simulink model "Polynomial_model_for_locked_state_1"  (R2025a)
settings: Solver=VariableStepAuto  StartTime=0.0  StopTime=10.0  RelTol=1e-3
values from neighbouring files (symbols this model uses):
  Divider_Controller = 0    [Close_Loop_ENOP_stable.m]
  IC1 = [0 0 0 0]    [Close_Loop_ENOP_stable.m]
  icp_offset = 0    [Close_Loop_ENOP_stable.m]
  inp = 1023    [Close_Loop_ENOP_stable.m]
  LSB_Dither = 1    [Close_Loop_ENOP_stable.m]
  M = 1024^2    (= 1048576)    [Close_Loop_ENOP_stable.m]
  Nint = 45    [Close_Loop_ENOP_stable.m]
libraries: dspobslib x5
settings Model: Creator=haoyang  LastModifiedBy=HaoyangShen

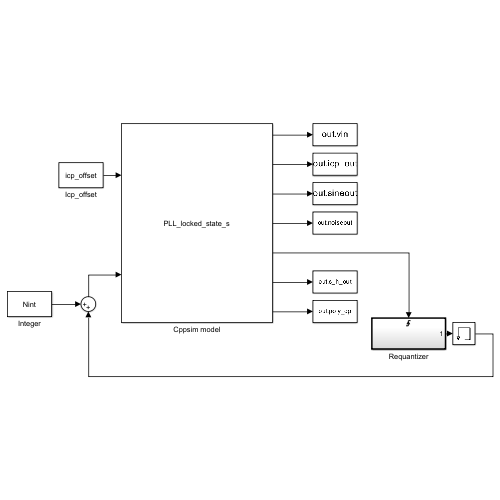
[thumbnail: Simulink's stored preview of the top-level diagram]
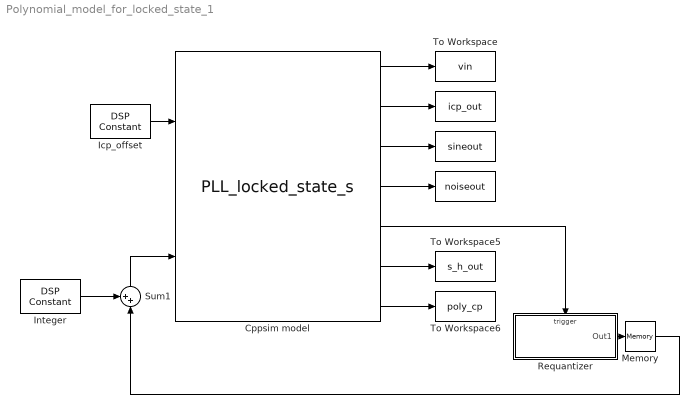
== system Polynomial_model_for_locked_state_1 ==
  " " : ToWorkspace  VariableName=icp_out  SampleTime=-1
  "  " : ToWorkspace  VariableName=sineout  SampleTime=-1
  "   " : ToWorkspace  VariableName=noiseout  SampleTime=-1
  Cppsim model : S-Function  FunctionName=PLL_locked_state_s  Parameters=Ts, pfd_freq, pfd_reset_delay, pfd_down_xdelay, icp, icp_error, icp_thermal_noise_up, icp_thermal_noise_down, icp_flicker_corner_freq_up, icp_flicker_corner_freq_down, s_and_h_en, fpole1, fzero, fgain, fpole2, vco_fc, vco_kv, vco_foffset, vco_noise_at_foffset, a0, a1, a2, a3, a4, a5, a6, a7, pre_gain, settle_sample  SFunctionDeploymentMode=off  EnableBusSupport=off
  Icp_offset : dspobslib/DSP Constant  Value=icp_offset  SampleMode=Discrete  discreteOutput=Sample-based (interpret vectors as 1-D)  continuousOutput=Sample-based  sampTime=-1  framePeriod=2  dataType=Inherit from 'Constant value'  isSigned=on  wordLen=16  udDataType=sfix(16)  fracBitsMode=Best precision  numFracBits=15  InterpretAs1D=-inf  Ts=-inf  FramebasedOutput=-inf
  Integer : dspobslib/DSP Constant  Value=Nint  SampleMode=Discrete  discreteOutput=Sample-based (interpret vectors as 1-D)  continuousOutput=Sample-based  sampTime=-1  framePeriod=2  dataType=Inherit from 'Constant value'  isSigned=on  wordLen=16  udDataType=sfix(16)  fracBitsMode=Best precision  numFracBits=15  InterpretAs1D=-inf  Ts=-inf  FramebasedOutput=-inf
  Memory : Memory
  Requantizer : Subsystem  TreatAsAtomicUnit=on
  Sum1 : Sum  Inputs=++|
  To Workspace : ToWorkspace  VariableName=vin  SampleTime=-1
  To Workspace5 : ToWorkspace  VariableName=s_h_out  SampleTime=-1
  To Workspace6 : ToWorkspace  VariableName=poly_cp  SampleTime=-1
  wires:
  Cppsim model/4 -> "   "/1
  Requantizer/1(Out1) -> Memory/1
  Integer/1 -> Sum1/1
  Cppsim model/3 -> "  "/1
  Icp_offset/1 -> Cppsim model/1
  Cppsim model/2 -> " "/1
  Cppsim model/1 -> To Workspace/1
  Memory/1 -> Sum1/2
  Sum1/1 -> Cppsim model/2
  Cppsim model/5 -> Requantizer/Trigger
  Cppsim model/6 -> To Workspace5/1
  Cppsim model/7 -> To Workspace6/1

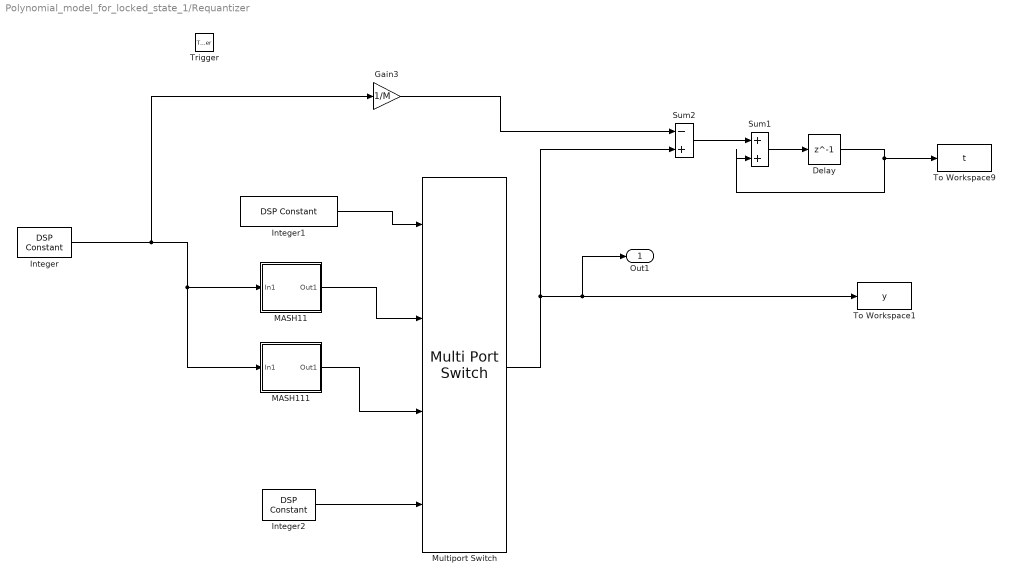
== system Polynomial_model_for_locked_state_1/Requantizer ==
  Trigger : TriggerPort  VariantControl=Variant
  Delay : Delay  DelayLength=1  InitialCondition=0
  Gain3 : Gain  Gain=1/M
  Integer : dspobslib/DSP Constant  Value=inp  SampleMode=Discrete  discreteOutput=Sample-based (interpret vectors as 1-D)  continuousOutput=Sample-based  sampTime=-1  framePeriod=2  dataType=Inherit from 'Constant value'  isSigned=on  wordLen=16  udDataType=sfix(16)  fracBitsMode=Best precision  numFracBits=15  InterpretAs1D=-inf  Ts=-inf  FramebasedOutput=-inf
  Integer1 : dspobslib/DSP Constant  Value=Divider_Controller  SampleMode=Discrete  discreteOutput=Sample-based (interpret vectors as 1-D)  continuousOutput=Sample-based  sampTime=-1  framePeriod=2  dataType=Inherit from 'Constant value'  isSigned=on  wordLen=16  udDataType=sfix(16)  fracBitsMode=Best precision  numFracBits=15  InterpretAs1D=-inf  Ts=-inf  FramebasedOutput=-inf
  Integer2 : dspobslib/DSP Constant  Value=0  SampleMode=Discrete  discreteOutput=Sample-based (interpret vectors as 1-D)  continuousOutput=Sample-based  sampTime=-1  framePeriod=2  dataType=Inherit from 'Constant value'  isSigned=on  wordLen=16  udDataType=sfix(16)  fracBitsMode=Best precision  numFracBits=15  InterpretAs1D=-inf  Ts=-inf  FramebasedOutput=-inf
  MASH11 : Subsystem
  MASH111 : Subsystem
  Multiport Switch : MultiPortSwitch  Inputs=2  DataPortForDefault=Additional data port  DiagnosticForDefault=None  SaturateOnIntegerOverflow=off  InputSameDT=off
  Sum1 : Sum  Inputs=++|
  Sum2 : Sum  Inputs=-+
  To Workspace1 : ToWorkspace  VariableName=y  SampleTime=-1
  To Workspace9 : ToWorkspace  VariableName=t  SampleTime=-1
  Out1 : Outport  VectorParamsAs1DForOutWhenUnconnected=off
  wires:
  Integer/1 -> Gain3/1, MASH111/1(In1), MASH11/1(In1)
  Gain3/1 -> Sum2/1
  Sum2/1 -> Sum1/1
  Sum1/1 -> Delay/1
  Delay/1 -> Sum1/2, To Workspace9/1
  Multiport Switch/1 -> Sum2/2, Out1/1, To Workspace1/1
  Integer1/1 -> Multiport Switch/1
  MASH11/1(Out1) -> Multiport Switch/2
  MASH111/1(Out1) -> Multiport Switch/3
  Integer2/1 -> Multiport Switch/4

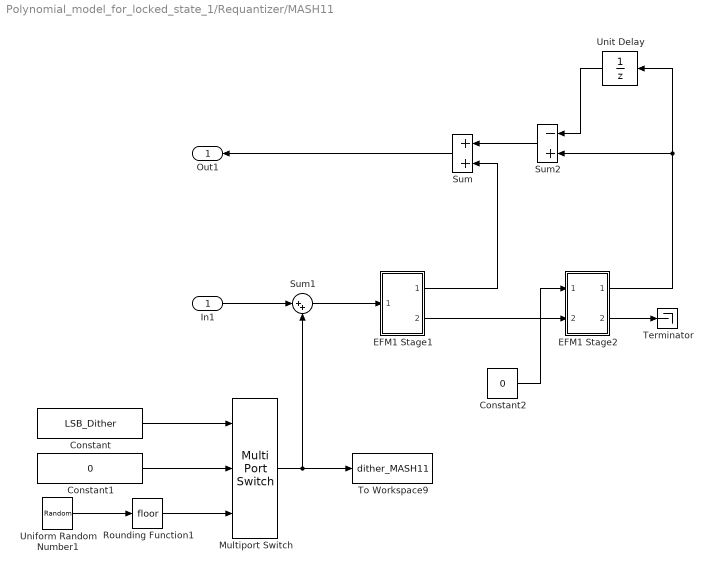
== system Polynomial_model_for_locked_state_1/Requantizer/MASH11 ==
  In1 : Inport
  Constant : Constant  Value=LSB_Dither  SampleTime=-1
  Constant1 : Constant  Value=0  SampleTime=-1
  Constant2 : Constant  Value=0  SampleTime=-1
  EFM1 Stage1 : Subsystem
  EFM1 Stage2 : Subsystem
  Multiport Switch : MultiPortSwitch  DataPortOrder=Specify indices  Inputs=2  DataPortIndices={0,1}  DiagnosticForDefault=None  SaturateOnIntegerOverflow=off  InputSameDT=off
  Rounding Function1 : Rounding
  Sum : Sum
  Sum1 : Sum  Inputs=|++
  Sum2 : Sum  Inputs=-+
  Terminator : Terminator
  To Workspace9 : ToWorkspace  VariableName=dither_MASH11  SampleTime=-1
  Uniform Random Number1 : UniformRandomNumber  Minimum=0  Maximum=2  Seed=101
  Unit Delay : UnitDelay  SampleTime=-1  HasFrameUpgradeWarning=on
  Out1 : Outport  VectorParamsAs1DForOutWhenUnconnected=off
  wires:
  EFM1 Stage1/1("Out1 ") -> Sum/2
  Rounding Function1/1 -> Multiport Switch/3
  Multiport Switch/1 -> Sum1/2, To Workspace9/1
  In1/1 -> Sum1/1
  Constant/1 -> Multiport Switch/1
  EFM1 Stage2/2(Out2) -> Terminator/1
  Constant1/1 -> Multiport Switch/2
  Unit Delay/1 -> Sum2/1
  Uniform Random Number1/1 -> Rounding Function1/1
  EFM1 Stage1/2(Out2) -> EFM1 Stage2/2(In1)
  Sum1/1 -> EFM1 Stage1/1(In1)
  EFM1 Stage2/1(Out1) -> Unit Delay/1, Sum2/2
  Sum/1 -> Out1/1
  Sum2/1 -> Sum/1
  Constant2/1 -> EFM1 Stage2/1(In2)

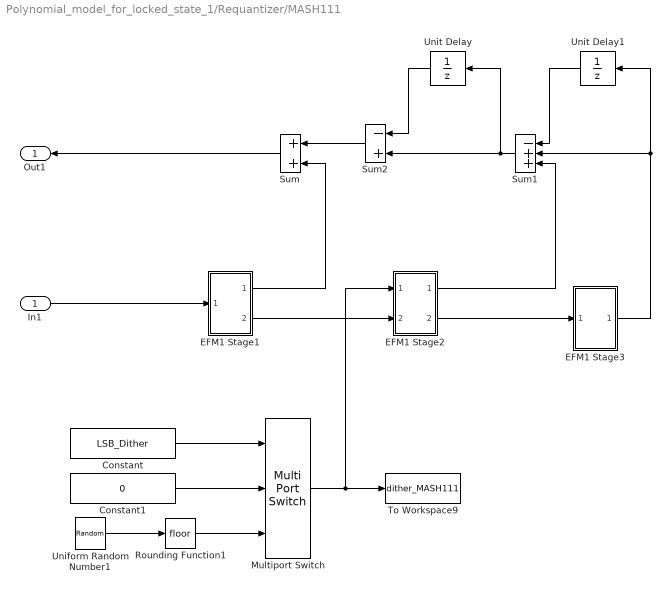
== system Polynomial_model_for_locked_state_1/Requantizer/MASH111 ==
  In1 : Inport
  Constant : Constant  Value=LSB_Dither  SampleTime=-1
  Constant1 : Constant  Value=0  SampleTime=-1
  EFM1 Stage1 : Subsystem
  EFM1 Stage2 : Subsystem
  EFM1 Stage3 : Subsystem
  Multiport Switch : MultiPortSwitch  DataPortOrder=Specify indices  Inputs=2  DataPortIndices={0,1}  DiagnosticForDefault=None  SaturateOnIntegerOverflow=off  InputSameDT=off
  Rounding Function1 : Rounding
  Sum : Sum
  Sum1 : Sum  Inputs=-++
  Sum2 : Sum  Inputs=-+
  To Workspace9 : ToWorkspace  VariableName=dither_MASH111  SampleTime=-1
  Uniform Random Number1 : UniformRandomNumber  Minimum=0  Maximum=2  Seed=101
  Unit Delay : UnitDelay  SampleTime=-1  HasFrameUpgradeWarning=on
  Unit Delay1 : UnitDelay  SampleTime=-1  HasFrameUpgradeWarning=on
  Out1 : Outport  VectorParamsAs1DForOutWhenUnconnected=off
  wires:
  Rounding Function1/1 -> Multiport Switch/3
  Constant1/1 -> Multiport Switch/2
  Sum2/1 -> Sum/1
  Multiport Switch/1 -> To Workspace9/1, EFM1 Stage2/1(In2)
  EFM1 Stage3/1(Out1) -> Unit Delay1/1, Sum1/2
  EFM1 Stage1/1("Out1 ") -> Sum/2
  Unit Delay/1 -> Sum2/1
  Uniform Random Number1/1 -> Rounding Function1/1
  Sum/1 -> Out1/1
  EFM1 Stage2/1(Out1) -> Sum1/3
  In1/1 -> EFM1 Stage1/1(In1)
  Unit Delay1/1 -> Sum1/1
  Constant/1 -> Multiport Switch/1
  Sum1/1 -> Unit Delay/1, Sum2/2
  EFM1 Stage1/2(Out2) -> EFM1 Stage2/2(In1)
  EFM1 Stage2/2(Out2) -> EFM1 Stage3/1(In2)

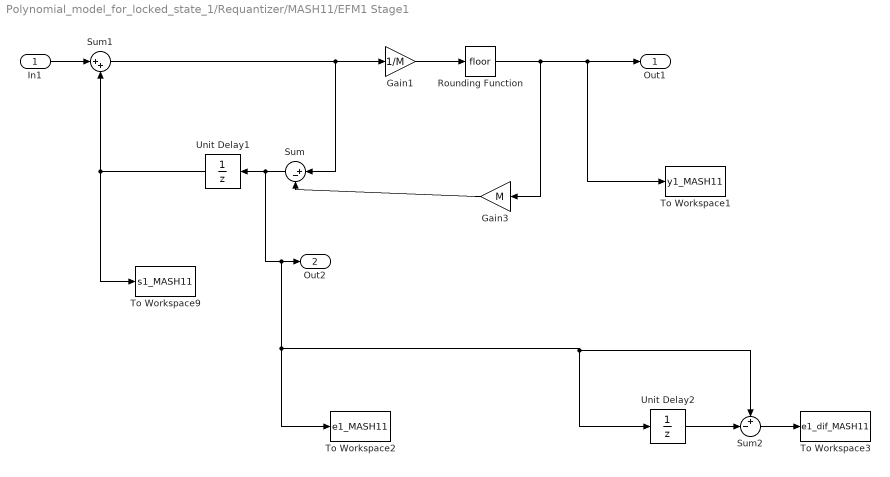
== system Polynomial_model_for_locked_state_1/Requantizer/MASH11/EFM1 Stage1 ==
  In1 : Inport
  Gain1 : Gain  Gain=1/M
  Gain3 : Gain  Gain=M
  Rounding Function : Rounding
  Sum : Sum  Inputs=|+-
  Sum1 : Sum  Inputs=|++
  Sum2 : Sum  Inputs=+-|
  To Workspace1 : ToWorkspace  VariableName=y1_MASH11  SampleTime=-1
  To Workspace2 : ToWorkspace  VariableName=e1_MASH11  SampleTime=-1
  To Workspace3 : ToWorkspace  VariableName=e1_dif_MASH11  SampleTime=-1
  To Workspace9 : ToWorkspace  VariableName=s1_MASH11  SampleTime=-1
  Unit Delay1 : UnitDelay  InitialCondition=IC1(1)  SampleTime=-1  HasFrameUpgradeWarning=on
  Unit Delay2 : UnitDelay  SampleTime=-1  HasFrameUpgradeWarning=on
  "Out1 " : Outport  VectorParamsAs1DForOutWhenUnconnected=off
  Out2 : Outport  Port=2  VectorParamsAs1DForOutWhenUnconnected=off
  wires:
  Sum1/1 -> Sum/1, Gain1/1
  Rounding Function/1 -> Gain3/1, To Workspace1/1, "Out1 "/1
  Gain3/1 -> Sum/2
  Gain1/1 -> Rounding Function/1
  In1/1 -> Sum1/1
  Unit Delay1/1 -> Sum1/2, To Workspace9/1
  Unit Delay2/1 -> Sum2/2
  Sum2/1 -> To Workspace3/1
  Sum/1 -> Unit Delay1/1, Sum2/1, Unit Delay2/1, To Workspace2/1, Out2/1

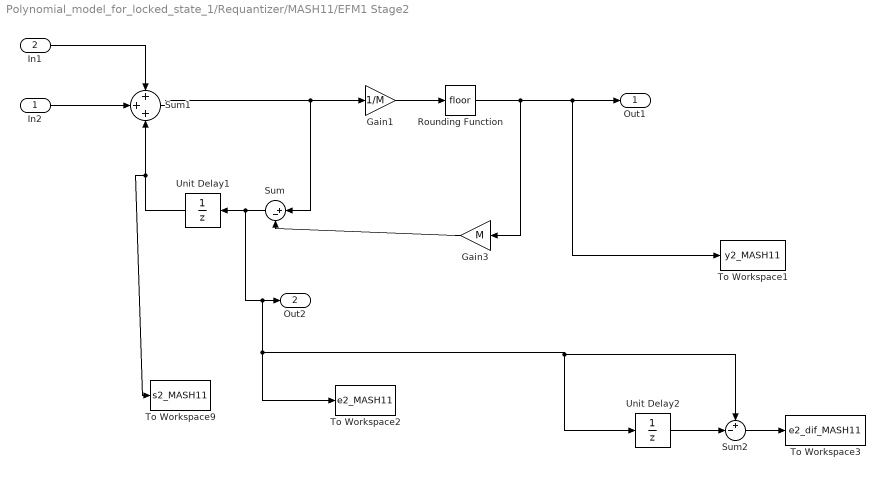
== system Polynomial_model_for_locked_state_1/Requantizer/MASH11/EFM1 Stage2 ==
  In2 : Inport
  In1 : Inport  Port=2
  Gain1 : Gain  Gain=1/M
  Gain3 : Gain  Gain=M
  Rounding Function : Rounding
  Sum : Sum  Inputs=|+-
  Sum1 : Sum  Inputs=+++
  Sum2 : Sum  Inputs=+-|
  To Workspace1 : ToWorkspace  VariableName=y2_MASH11  SampleTime=-1
  To Workspace2 : ToWorkspace  VariableName=e2_MASH11  SampleTime=-1
  To Workspace3 : ToWorkspace  VariableName=e2_dif_MASH11  SampleTime=-1
  To Workspace9 : ToWorkspace  VariableName=s2_MASH11  SampleTime=-1
  Unit Delay1 : UnitDelay  InitialCondition=IC1(2)  SampleTime=-1  HasFrameUpgradeWarning=on
  Unit Delay2 : UnitDelay  SampleTime=-1  HasFrameUpgradeWarning=on
  Out1 : Outport  VectorParamsAs1DForOutWhenUnconnected=off
  Out2 : Outport  Port=2  VectorParamsAs1DForOutWhenUnconnected=off
  wires:
  Sum1/1 -> Sum/1, Gain1/1
  Rounding Function/1 -> Gain3/1, To Workspace1/1, Out1/1
  Gain3/1 -> Sum/2
  Gain1/1 -> Rounding Function/1
  In1/1 -> Sum1/1
  Unit Delay1/1 -> Sum1/3, To Workspace9/1
  In2/1 -> Sum1/2
  Sum2/1 -> To Workspace3/1
  Sum/1 -> Unit Delay1/1, Sum2/1, Unit Delay2/1, To Workspace2/1, Out2/1
  Unit Delay2/1 -> Sum2/2

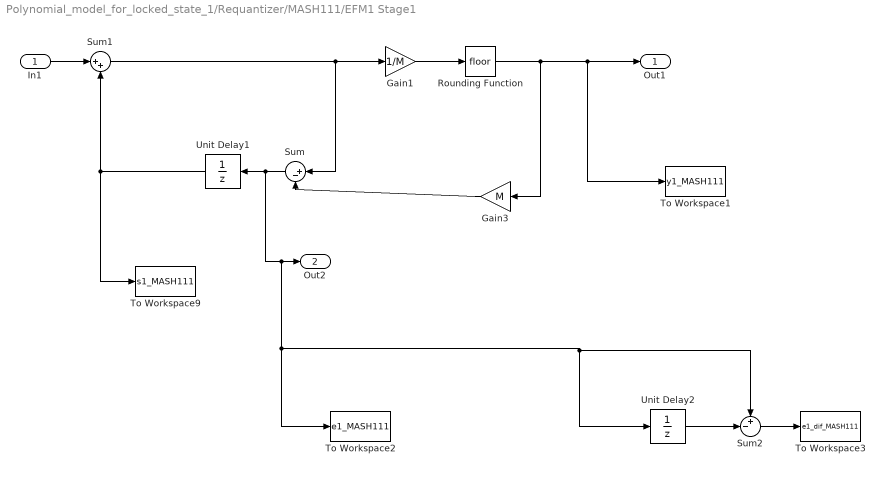
== system Polynomial_model_for_locked_state_1/Requantizer/MASH111/EFM1 Stage1 ==
  In1 : Inport
  Gain1 : Gain  Gain=1/M
  Gain3 : Gain  Gain=M
  Rounding Function : Rounding
  Sum : Sum  Inputs=|+-
  Sum1 : Sum  Inputs=|++
  Sum2 : Sum  Inputs=+-|
  To Workspace1 : ToWorkspace  VariableName=y1_MASH111  SampleTime=-1
  To Workspace2 : ToWorkspace  VariableName=e1_MASH111  SampleTime=-1
  To Workspace3 : ToWorkspace  VariableName=e1_dif_MASH111  SampleTime=-1
  To Workspace9 : ToWorkspace  VariableName=s1_MASH111  SampleTime=-1
  Unit Delay1 : UnitDelay  InitialCondition=IC1(1)  SampleTime=-1  HasFrameUpgradeWarning=on
  Unit Delay2 : UnitDelay  SampleTime=-1  HasFrameUpgradeWarning=on
  "Out1 " : Outport  VectorParamsAs1DForOutWhenUnconnected=off
  Out2 : Outport  Port=2  VectorParamsAs1DForOutWhenUnconnected=off
  wires:
  Sum1/1 -> Sum/1, Gain1/1
  Rounding Function/1 -> Gain3/1, To Workspace1/1, "Out1 "/1
  Gain3/1 -> Sum/2
  Gain1/1 -> Rounding Function/1
  In1/1 -> Sum1/1
  Unit Delay1/1 -> Sum1/2, To Workspace9/1
  Unit Delay2/1 -> Sum2/2
  Sum2/1 -> To Workspace3/1
  Sum/1 -> Unit Delay1/1, Sum2/1, Unit Delay2/1, To Workspace2/1, Out2/1

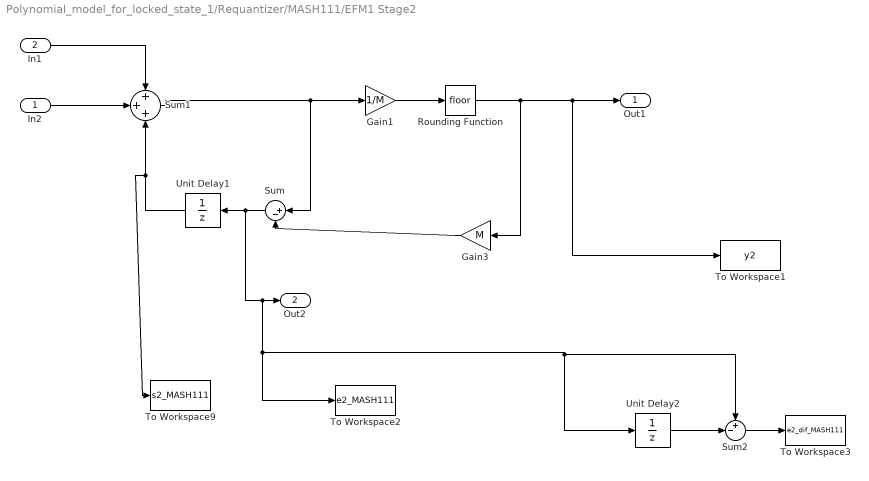
== system Polynomial_model_for_locked_state_1/Requantizer/MASH111/EFM1 Stage2 ==
  In2 : Inport
  In1 : Inport  Port=2
  Gain1 : Gain  Gain=1/M
  Gain3 : Gain  Gain=M
  Rounding Function : Rounding
  Sum : Sum  Inputs=|+-
  Sum1 : Sum  Inputs=+++
  Sum2 : Sum  Inputs=+-|
  To Workspace1 : ToWorkspace  VariableName=y2  SampleTime=-1
  To Workspace2 : ToWorkspace  VariableName=e2_MASH111  SampleTime=-1
  To Workspace3 : ToWorkspace  VariableName=e2_dif_MASH111  SampleTime=-1
  To Workspace9 : ToWorkspace  VariableName=s2_MASH111  SampleTime=-1
  Unit Delay1 : UnitDelay  InitialCondition=IC1(2)  SampleTime=-1  HasFrameUpgradeWarning=on
  Unit Delay2 : UnitDelay  SampleTime=-1  HasFrameUpgradeWarning=on
  Out1 : Outport  VectorParamsAs1DForOutWhenUnconnected=off
  Out2 : Outport  Port=2  VectorParamsAs1DForOutWhenUnconnected=off
  wires:
  Sum1/1 -> Sum/1, Gain1/1
  Rounding Function/1 -> Gain3/1, To Workspace1/1, Out1/1
  Gain3/1 -> Sum/2
  Gain1/1 -> Rounding Function/1
  In1/1 -> Sum1/1
  Unit Delay1/1 -> Sum1/3, To Workspace9/1
  In2/1 -> Sum1/2
  Sum2/1 -> To Workspace3/1
  Sum/1 -> Unit Delay1/1, Sum2/1, Unit Delay2/1, To Workspace2/1, Out2/1
  Unit Delay2/1 -> Sum2/2

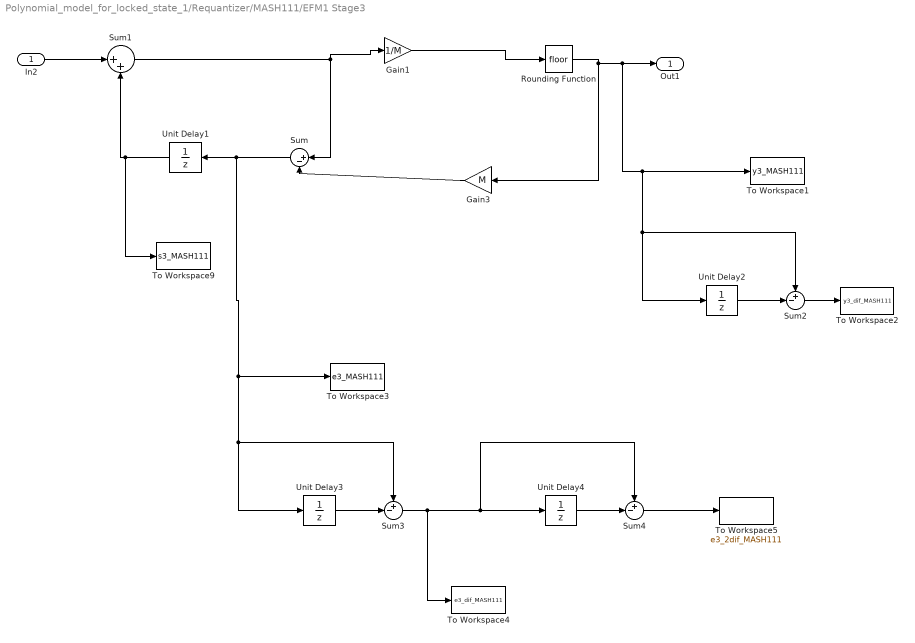
== system Polynomial_model_for_locked_state_1/Requantizer/MASH111/EFM1 Stage3 ==
  In2 : Inport
  Gain1 : Gain  Gain=1/M
  Gain3 : Gain  Gain=M
  Rounding Function : Rounding
  Sum : Sum  Inputs=|+-
  Sum1 : Sum  Inputs=|++
  Sum2 : Sum  Inputs=+-|
  Sum3 : Sum  Inputs=+-|
  Sum4 : Sum  Inputs=+-|
  To Workspace1 : ToWorkspace  VariableName=y3_MASH111  SampleTime=-1
  To Workspace2 : ToWorkspace  VariableName=y3_dif_MASH111  SampleTime=-1
  To Workspace3 : ToWorkspace  VariableName=e3_MASH111  SampleTime=-1
  To Workspace4 : ToWorkspace  VariableName=e3_dif_MASH111  SampleTime=-1
  To Workspace5 : ToWorkspace  VariableName=e3_2dif_MASH111  SampleTime=-1
  To Workspace9 : ToWorkspace  VariableName=s3_MASH111  SampleTime=-1
  Unit Delay1 : UnitDelay  InitialCondition=IC1(3)  SampleTime=-1  HasFrameUpgradeWarning=on
  Unit Delay2 : UnitDelay  SampleTime=-1  HasFrameUpgradeWarning=on
  Unit Delay3 : UnitDelay  SampleTime=-1  HasFrameUpgradeWarning=on
  Unit Delay4 : UnitDelay  SampleTime=-1  HasFrameUpgradeWarning=on
  Out1 : Outport  VectorParamsAs1DForOutWhenUnconnected=off
  wires:
  Rounding Function/1 -> Gain3/1, Sum2/1, Unit Delay2/1, To Workspace1/1, Out1/1
  Gain3/1 -> Sum/2
  Sum1/1 -> Gain1/1, Sum/1
  In2/1 -> Sum1/1
  Gain1/1 -> Rounding Function/1
  Unit Delay1/1 -> Sum1/2, To Workspace9/1
  Unit Delay2/1 -> Sum2/2
  Sum2/1 -> To Workspace2/1
  Unit Delay3/1 -> Sum3/2
  Sum/1 -> Unit Delay1/1, Sum3/1, Unit Delay3/1, To Workspace3/1
  Sum3/1 -> Sum4/1, Unit Delay4/1, To Workspace4/1
  Unit Delay4/1 -> Sum4/2
  Sum4/1 -> To Workspace5/1
